simulink model "Mdl_Speed"  (R2024b)
settings: Solver=FixedStepDiscrete  StartTime=0.0  StopTime=10.0  FixedStep=0.1  RelTol=1e-3  EnableMultiTasking=on
values from neighbouring files (symbols this model uses):
  AI_TEMP_ADC_COUNT_1586 = mpt.Parameter    [Mdl_Speed_lookup.m]
  AI_TEMP_ADC_COUNT_1727 = mpt.Parameter    [Mdl_Speed_lookup.m]
  AI_TEMP_ADC_COUNT_1792 = mpt.Parameter    [Mdl_Speed_lookup.m]
  AI_TEMP_ADC_COUNT_1891 = mpt.Parameter    [Mdl_Speed_lookup.m]
  C_ADR = mpt.Parameter    [Mdl_Speed_lookup.m]
  C_CANADA = mpt.Parameter    [Mdl_Speed_lookup.m]
  C_EUROPE = mpt.Parameter    [Mdl_Speed_lookup.m]
  C_KOREA = mpt.Parameter    [Mdl_Speed_lookup.m]
  C_MEXICO = mpt.Parameter    [Mdl_Speed_lookup.m]
  C_UK = mpt.Parameter    [Mdl_Speed_lookup.m]
  C_USA = mpt.Parameter    [Mdl_Speed_lookup.m]
  eSP_ADR = mpt.Parameter    [Speed_Table_Type_param.m]
  eSP_CANADA = mpt.Parameter    [Speed_Table_Type_param.m]
  eSP_ECE = mpt.Parameter    [Speed_Table_Type_param.m]
  eSP_EUROPE = mpt.Parameter    [Speed_Table_Type_param.m]
  eSP_KOREA_FMVSS = mpt.Parameter    [Speed_Table_Type_param.m]
  eSP_KOREA_UN_R = mpt.Parameter    [Speed_Table_Type_param.m]
  eSP_MEXICO_FMVSS = mpt.Parameter    [Speed_Table_Type_param.m]
  eSP_MEXICO_UN_R = mpt.Parameter    [Speed_Table_Type_param.m]
  eSP_UK = mpt.Parameter    [Speed_Table_Type_param.m]
  eSP_USA = mpt.Parameter    [Speed_Table_Type_param.m]
  INDEX_MCUID0262 = mpt.Parameter    [Mdl_Speed_lookup.m]
  INDEX_MCUID0263 = mpt.Parameter    [Mdl_Speed_lookup.m]
  Initial_data = mpt.Parameter    [Mdl_Speed_lookup.m]
  MCUID0809 = mpt.Parameter    [Mdl_Speed_DD.m]
  MCUID0810 = mpt.Parameter    [Mdl_Speed_DD.m]
  MCUID_MAX_VAL = mpt.Parameter    [Mdl_Speed_lookup.m]
  MIN_SPEED_VALUE = mpt.Parameter    [Mdl_Speed_lookup.m]
  RESOLUTION_VAL_100 = mpt.Parameter    [Mdl_Speed_lookup.m]
  RESOLUTION_VAL_103 = mpt.Parameter    [Mdl_Speed_lookup.m]
  RESOLUTION_VAL_50 = mpt.Parameter    [Mdl_Speed_lookup.m]
  RESOLUTION_VAL_64 = mpt.Parameter    [Mdl_Speed_lookup.m]
  RESOLUTION_VAL_MINUS_100 = mpt.Parameter    [Mdl_Speed_lookup.m]
  SPEED_AVG_REF = mpt.Parameter    [Mdl_Speed_lookup.m]
  SPEED_CHECK_VALUE_ONE = mpt.Parameter    [Mdl_Speed_lookup.m]
  SPEED_UPDATE_0_28S = mpt.Parameter    [Mdl_Speed_lookup.m]
  SPEED_UPDATE_0_5S = mpt.Parameter    [Mdl_Speed_lookup.m]
  SPEED_UPDATE_1_5S = mpt.Parameter    [Mdl_Speed_lookup.m]
  SPEED_UPDATE_1S = mpt.Parameter    [Mdl_Speed_lookup.m]
  SPEED_ZERO = mpt.Parameter    [Mdl_Speed_lookup.m]
  VAL_ONE = mpt.Parameter    [Mdl_Speed_lookup.m]
  VAL_ZERO = mpt.Parameter    [Mdl_Speed_lookup.m]
undefined symbols (not defined in the file or in its folder): Arr_u8_100_type_instance, Arr_u8_1024_type_instance, Arr_u8_10_type_instance, Arr_u8_128_type_instance, Arr_u8_16_type_instance, Arr_u8_17_type_instance, Arr_u8_2048_type_instance, Arr_u8_256_type_instance, Arr_u8_32_type_instance, Arr_u8_3_type_instance, Arr_u8_46_type_instance, Arr_u8_48_type_instance, Arr_u8_61_type_instance, Arr_u8_64_type_instance, Arr_u8_8_type_instance, Arr_u8_9_type_instance, CLUSTER_ACTIVE, eIO_ADC_AI_TEMP_RTC, eSIGNAL_MISSING, eSIGNAL_NEVER_RECEIVED, eVehicleSpeedABSIn, IgnOff, IgnOn, IoHwAb_AdcSignalIdType_type_instance, IoHwAb_ErrorType_type_instance, pJustRcvdStatus, RxCan_SignalClearJustRcvdStatus, RxCan_SignalGetJustRcvdStatus, RxCan_SignalInvalidProcessingControl, RxCan_SignalMissingProcessingControl, RxCan_SignalNRProcessingControl, SignalId, SPEED_MAX_RESOLUTION, Status, tRxSignalId_type_instance, tRxSignalJustRcvdStatus_type_instance, tRxSignalStatus_type_instance
libraries: simulink x9
(part 1 of 3)
settings Model: Creator=AELANGO6  LastModifiedBy=AELANGO6
settings DataIOCC: SaveOutput=off
settings OptimizationCC: DefaultParameterBehavior=Inlined  EnhancedBackFolding=on  PassReuseOutputArgsAs=Individual arguments  ZeroExternalMemoryAtStartup=off  ZeroInternalMemoryAtStartup=off  MaxStackSize=750  OptimizeBlockOrder=speed  DifferentSizesBufferReuse=on  OptimizationCustomize=off  EfficientTunableParamExpr=on
settings DebuggingCC: ParameterTunabilityLossMsg=error
settings SFSimCC: MATLABDynamicMemAlloc=off
settings RTWCC: Description=AUTOSAR  SystemTargetFile=autosar.tlc  GenCodeOnly=on  TemplateMakefile=ert_default_tmf  PortableWordSizes=on  DataTypeReplacement=CDataTypesFixedWidth
settings CodeAppCC: ForceParamTrailComments=on  IgnoreCustomStorageClasses=off  OperatorAnnotations=on  SimulinkDataObjDesc=on  SFDataObjDesc=on  InsertBlockDesc=on
settings STFCustomTargetCC: TargetLangStandard=C99 (ISO)  MultiwordLength=256  ParMdlRefBuildCompliant=on  CompOptLevelCompliant=on  IncludeMdlTerminateFcn=off  CombineOutputUpdateFcns=on  SuppressErrorStatus=on  ERTCustomFileBanners=on  SupportNonFinite=off  SupportComplex=off  SupportContinuousTime=off  SupportNonInlinedSFcns=off  RemoveResetFunc=on  ParenthesesLevel=Maximum  CastingMode=Standards  MATLABClassNameForMDSCustomization=Simulink.SoftwareTarget.ERTCustomization  AutosarCompliant=on  UseToolchainInfoCompliant=on  LookupTableObjectStructAxisOrder=2,1,3,4,...  LUTObjectStructOrderEvenSpacing=Size,Table,Breakpoints  SystemTargetFile=autosar.tlc
settings ERTTargetCC: TargetLangStandard=C99 (ISO)  ConcurrentExecutionCompliant=off  IncludeMdlTerminateFcn=off  SuppressErrorStatus=on  SupportNonFinite=off  SupportComplex=off  ParenthesesLevel=Maximum  CastingMode=Standards  ModelStepFunctionPrototypeControlCompliant=off  CPPClassGenCompliant=off  AutosarCompliant=on  LookupTableObjectStructAxisOrder=2,1,3,4,...  LUTObjectStructOrderEvenSpacing=Size,Table,Breakpoints  ERTCustomFileTemplate=example_file_process.tlc  ERTFilePackagingFormat=CompactWithDataFile  BooleanTrueId=TRUE  BooleanFalseId=FALSE

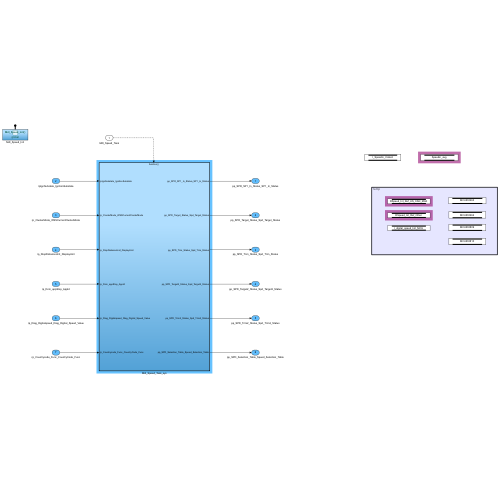
[thumbnail: Simulink's stored preview of the top-level diagram]
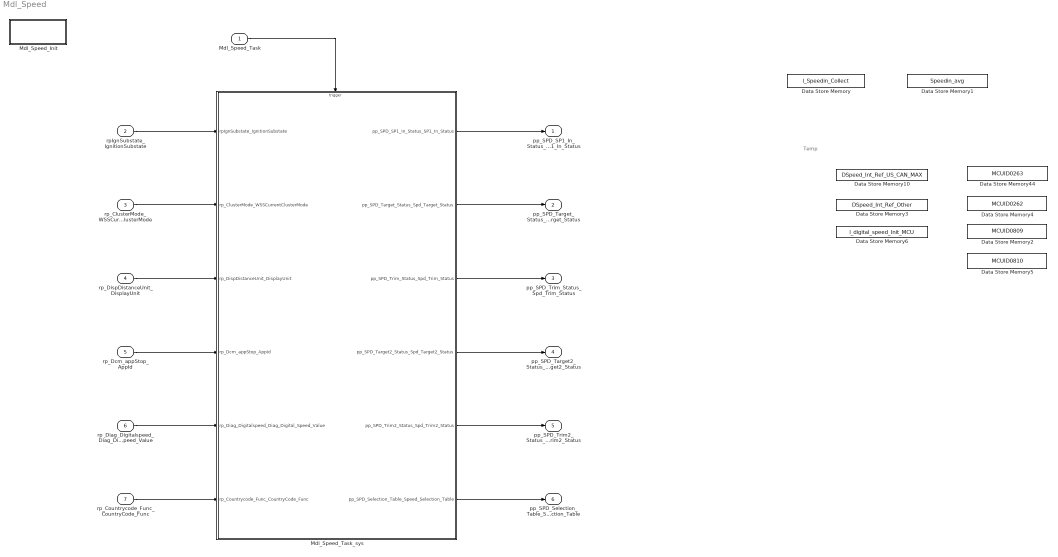
== system Mdl_Speed ==
  note: Temp
  Mdl_Speed_Task : Inport  SampleTime=0.1  OutputFunctionCall=on
  rpIgnSubstate_IgnitionSubstate : Inport  Port=2  OutDataTypeStr=IgntionSubstateType  PortDimensions=1
  rp_ClusterMode_WSSCurrentClusterMode : Inport  Port=3  OutDataTypeStr=ClusterModes  PortDimensions=1
  rp_DispDistanceUnit_DisplayUnit : Inport  Port=4  OutDataTypeStr=uint8  PortDimensions=1
  rp_Dcm_appStop_AppId : Inport  Port=5  OutDataTypeStr=IOCtrl_Type  PortDimensions=1
  rp_Diag_Digitalspeed_Diag_Digital_Speed_Value : Inport  Port=6  OutDataTypeStr=uint16  PortDimensions=1
  rp_Countrycode_Func_CountryCode_Func : Inport  Port=7  OutDataTypeStr=CountryCode_FuncType  PortDimensions=1
  Data Store Memory : DataStoreMemory  DataStoreName=l_Speedin_Collect  ReadBeforeWriteMsg=warning  WriteAfterWriteMsg=warning  WriteAfterReadMsg=warning  ShowAdditionalParam=off  OutDataTypeStr=uint32
  Data Store Memory1 : DataStoreMemory  DataStoreName=Speedin_avg  ReadBeforeWriteMsg=warning  WriteAfterWriteMsg=warning  WriteAfterReadMsg=warning  ShowAdditionalParam=off  OutDataTypeStr=uint16
  Data Store Memory10 : DataStoreMemory  DataStoreName=DSpeed_Int_Ref_US_CAN_MAX  ReadBeforeWriteMsg=warning  WriteAfterWriteMsg=warning  WriteAfterReadMsg=warning  InitialValue=Initial_data  ShowAdditionalParam=off  OutDataTypeStr=uint16  Dimensions=21
  Data Store Memory2 : DataStoreMemory  DataStoreName=MCUID0809  ReadBeforeWriteMsg=warning  WriteAfterWriteMsg=warning  WriteAfterReadMsg=warning  InitialValue=VAL_ZERO  ShowAdditionalParam=off  OutDataTypeStr=uint8
  Data Store Memory3 : DataStoreMemory  DataStoreName=DSpeed_Int_Ref_Other  ReadBeforeWriteMsg=warning  WriteAfterWriteMsg=warning  WriteAfterReadMsg=warning  InitialValue=Initial_data  ShowAdditionalParam=off  OutDataTypeStr=uint16  Dimensions=21
  Data Store Memory4 : DataStoreMemory  DataStoreName=MCUID0262  ReadBeforeWriteMsg=warning  WriteAfterWriteMsg=warning  WriteAfterReadMsg=warning  InitialValue=CNVM_MCUID0262_DEFAULT_VAL  ShowAdditionalParam=off  OutDataTypeStr=uint16
  Data Store Memory44 : DataStoreMemory  DataStoreName=MCUID0263  ReadBeforeWriteMsg=warning  WriteAfterWriteMsg=warning  WriteAfterReadMsg=warning  InitialValue=CNVM_MCUID0263_DEFAULT_VAL  ShowAdditionalParam=off  OutDataTypeStr=uint16
  Data Store Memory5 : DataStoreMemory  DataStoreName=MCUID0810  ReadBeforeWriteMsg=warning  WriteAfterWriteMsg=warning  WriteAfterReadMsg=warning  InitialValue=VAL_ONE  ShowAdditionalParam=off  OutDataTypeStr=uint8
  Data Store Memory6 : DataStoreMemory  DataStoreName=l_digital_speed_Init_MCU  ReadBeforeWriteMsg=warning  WriteAfterWriteMsg=warning  WriteAfterReadMsg=warning  InitialValue=VAL_ZERO  ShowAdditionalParam=off  OutDataTypeStr=uint8
  Mdl_Speed_Init : Subsystem  TreatAsAtomicUnit=on
  Mdl_Speed_Task_sys : Subsystem  TreatAsAtomicUnit=on
  pp_SPD_SP1_In_Status_SP1_In_Status : Outport  OutDataTypeStr=uint16
  pp_SPD_Target_Status_Spd_Target_Status : Outport  Port=2  OutDataTypeStr=uint16
  pp_SPD_Trim_Status_Spd_Trim_Status : Outport  Port=3  OutDataTypeStr=uint16
  pp_SPD_Target2_Status_Spd_Target2_Status : Outport  Port=4  OutDataTypeStr=uint16
  pp_SPD_Trim2_Status_Spd_Trim2_Status : Outport  Port=5  OutDataTypeStr=uint16
  pp_SPD_Selection_Table_Speed_Selection_Table : Outport  Port=6  OutDataTypeStr=uint8
  wires:
  rp_Countrycode_Func_CountryCode_Func/1 -> Mdl_Speed_Task_sys/6(rp_Countrycode_Func_CountryCode_Func)
  rpIgnSubstate_IgnitionSubstate/1 -> Mdl_Speed_Task_sys/1(rpIgnSubstate_IgnitionSubstate)
  Mdl_Speed_Task/1 -> Mdl_Speed_Task_sys/Trigger
  rp_ClusterMode_WSSCurrentClusterMode/1 -> Mdl_Speed_Task_sys/2(rp_ClusterMode_WSSCurrentClusterMode)
  rp_DispDistanceUnit_DisplayUnit/1 -> Mdl_Speed_Task_sys/3(rp_DispDistanceUnit_DisplayUnit)
  rp_Dcm_appStop_AppId/1 -> Mdl_Speed_Task_sys/4(rp_Dcm_appStop_AppId)
  rp_Diag_Digitalspeed_Diag_Digital_Speed_Value/1 -> Mdl_Speed_Task_sys/5(rp_Diag_Digitalspeed_Diag_Digital_Speed_Value)
  Mdl_Speed_Task_sys/1(pp_SPD_SP1_In_Status_SP1_In_Status) -> pp_SPD_SP1_In_Status_SP1_In_Status/1
  Mdl_Speed_Task_sys/2(pp_SPD_Target_Status_Spd_Target_Status) -> pp_SPD_Target_Status_Spd_Target_Status/1
  Mdl_Speed_Task_sys/3(pp_SPD_Trim_Status_Spd_Trim_Status) -> pp_SPD_Trim_Status_Spd_Trim_Status/1
  Mdl_Speed_Task_sys/4(pp_SPD_Target2_Status_Spd_Target2_Status) -> pp_SPD_Target2_Status_Spd_Target2_Status/1
  Mdl_Speed_Task_sys/5(pp_SPD_Trim2_Status_Spd_Trim2_Status) -> pp_SPD_Trim2_Status_Spd_Trim2_Status/1
  Mdl_Speed_Task_sys/6(pp_SPD_Selection_Table_Speed_Selection_Table) -> pp_SPD_Selection_Table_Speed_Selection_Table/1

== system Mdl_Speed/Mdl_Speed_Init ==
  Mdl_Speed_Init : TriggerPort  TriggerType=function-call  IsSimulinkFunction=on  FunctionName=Mdl_Speed_Init  VariantControl=(inherit)

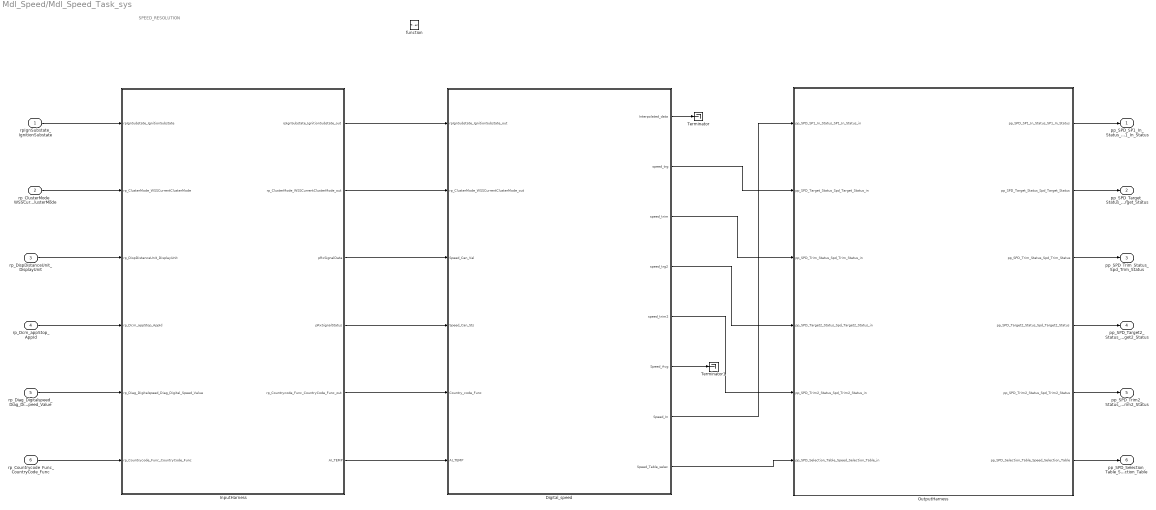
== system Mdl_Speed/Mdl_Speed_Task_sys ==
  note: SPEED_RESOLUTION
  rpIgnSubstate_IgnitionSubstate : Inport  OutDataTypeStr=IgntionSubstateType  PortDimensions=1
  rp_ClusterMode_WSSCurrentClusterMode : Inport  Port=2  OutDataTypeStr=ClusterModes  PortDimensions=1
  rp_DispDistanceUnit_DisplayUnit : Inport  Port=3  OutDataTypeStr=uint8  PortDimensions=1
  rp_Dcm_appStop_AppId : Inport  Port=4  OutDataTypeStr=IOCtrl_Type  PortDimensions=1
  rp_Diag_Digitalspeed_Diag_Digital_Speed_Value : Inport  Port=5  OutDataTypeStr=uint16  PortDimensions=1
  rp_Countrycode_Func_CountryCode_Func : Inport  Port=6  OutDataTypeStr=CountryCode_FuncType  PortDimensions=1
  function : TriggerPort  TriggerType=function-call  VariantControl=(inherit)  SampleTimeType=periodic  SampleTime=-1
  Digital_speed : Subsystem
  InputHarness : Subsystem  Variant=on
  OutputHarness : Subsystem  Variant=on
  Terminator : Terminator
  Terminator1 : Terminator
  pp_SPD_SP1_In_Status_SP1_In_Status : Outport  OutDataTypeStr=uint16  PortDimensions=1
  pp_SPD_Target_Status_Spd_Target_Status : Outport  Port=2  OutDataTypeStr=uint16  PortDimensions=1
  pp_SPD_Trim_Status_Spd_Trim_Status : Outport  Port=3  OutDataTypeStr=uint16  PortDimensions=1
  pp_SPD_Target2_Status_Spd_Target2_Status : Outport  Port=4  OutDataTypeStr=uint16  PortDimensions=1
  pp_SPD_Trim2_Status_Spd_Trim2_Status : Outport  Port=5  OutDataTypeStr=uint16  PortDimensions=1
  pp_SPD_Selection_Table_Speed_Selection_Table : Outport  Port=6  OutDataTypeStr=uint8  PortDimensions=1
  wires:
  rp_Countrycode_Func_CountryCode_Func/1 -> InputHarness/6(rp_Countrycode_Func_CountryCode_Func)
  rpIgnSubstate_IgnitionSubstate/1 -> InputHarness/1(rpIgnSubstate_IgnitionSubstate)
  rp_ClusterMode_WSSCurrentClusterMode/1 -> InputHarness/2(rp_ClusterMode_WSSCurrentClusterMode)
  rp_DispDistanceUnit_DisplayUnit/1 -> InputHarness/3(rp_DispDistanceUnit_DisplayUnit)
  rp_Dcm_appStop_AppId/1 -> InputHarness/4(rp_Dcm_appStop_AppId)
  rp_Diag_Digitalspeed_Diag_Digital_Speed_Value/1 -> InputHarness/5(rp_Diag_Digitalspeed_Diag_Digital_Speed_Value)
  OutputHarness/1(pp_SPD_SP1_In_Status_SP1_In_Status) -> pp_SPD_SP1_In_Status_SP1_In_Status/1
  OutputHarness/2(pp_SPD_Target_Status_Spd_Target_Status) -> pp_SPD_Target_Status_Spd_Target_Status/1
  OutputHarness/3(pp_SPD_Trim_Status_Spd_Trim_Status) -> pp_SPD_Trim_Status_Spd_Trim_Status/1
  OutputHarness/4(pp_SPD_Target2_Status_Spd_Target2_Status) -> pp_SPD_Target2_Status_Spd_Target2_Status/1
  OutputHarness/5(pp_SPD_Trim2_Status_Spd_Trim2_Status) -> pp_SPD_Trim2_Status_Spd_Trim2_Status/1
  OutputHarness/6(pp_SPD_Selection_Table_Speed_Selection_Table) -> pp_SPD_Selection_Table_Speed_Selection_Table/1
  InputHarness/1(rpIgnSubstate_IgnitionSubstate_out) -> Digital_speed/1(rpIgnSubstate_IgnitionSubstate_out)
  InputHarness/2(rp_ClusterMode_WSSCurrentClusterMode_out) -> Digital_speed/2(rp_ClusterMode_WSSCurrentClusterMode_out)
  InputHarness/3(pRxSignalData) -> Digital_speed/3(Speed_Can_Val)
  InputHarness/4(pRxSignalStatus) -> Digital_speed/4(Speed_Can_Sts)
  InputHarness/6(AI_TEMP) -> Digital_speed/6(AI_TEMP)
  InputHarness/5(rp_Countrycode_Func_CountryCode_Func_out) -> Digital_speed/5(Country_code_Func)
  Digital_speed/2(speed_trg) -> OutputHarness/2(pp_SPD_Target_Status_Spd_Target_Status_in)
  Digital_speed/1(Interpolated_data) -> Terminator/1
  Digital_speed/6(Speed_Avg) -> Terminator1/1
  Digital_speed/3(speed_trim) -> OutputHarness/3(pp_SPD_Trim_Status_Spd_Trim_Status_in)
  Digital_speed/4(speed_trg2) -> OutputHarness/4(pp_SPD_Target2_Status_Spd_Target2_Status_in)
  Digital_speed/5(speed_trim2) -> OutputHarness/5(pp_SPD_Trim2_Status_Spd_Trim2_Status_in)
  Digital_speed/7(Speed_In) -> OutputHarness/1(pp_SPD_SP1_In_Status_SP1_In_Status_in)
  Digital_speed/8(Speed_Table_selec) -> OutputHarness/6(pp_SPD_Selection_Table_Speed_Selection_Table_in)

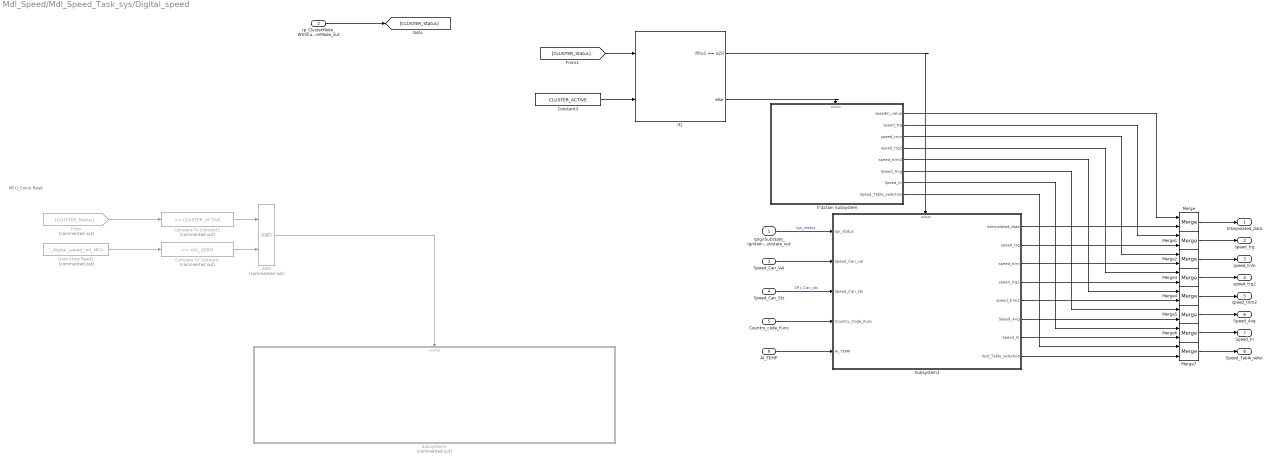
== system Mdl_Speed/Mdl_Speed_Task_sys/Digital_speed ==
  note: MCU_Const Read
  rpIgnSubstate_IgnitionSubstate_out : Inport  OutDataTypeStr=IgntionSubstateType  PortDimensions=1
  rp_ClusterMode_WSSCurrentClusterMode_out : Inport  Port=2
  Speed_Can_Val : Inport  Port=3  OutDataTypeStr=uint8
  Speed_Can_Sts : Inport  Port=4  OutDataTypeStr=uint8
  Country_code_Func : Inport  Port=5  OutDataTypeStr=uint8
  AI_TEMP : Inport  Port=6
  AND : Logic  Commented=on  AllPortsSameDT=off  OutDataTypeStr=boolean
  Compare To Constant : simulink/Logic and Bit Operations/Compare To Constant  Commented=on  relop===  const=VAL_ZERO  OutDataTypeStr=boolean
  Compare To Constant1 : simulink/Logic and Bit Operations/Compare To Constant  Commented=on  relop===  const=CLUSTER_ACTIVE  OutDataTypeStr=boolean
  Constant3 : Constant  Value=CLUSTER_ACTIVE
  Data Store Read2 : DataStoreRead  Commented=on  DataStoreName=l_digital_speed_Init_MCU  IndexOptions=Index vector (dialog)  Indices=1  OutputSizes=1
  From : From  Commented=on  GotoTag=CLUSTER_Status
  If Action Subsystem : Subsystem  TreatAsAtomicUnit=on
  If1 : If  NumInputs=2  IfExpression=(u1 == u2)
  Merge{,1..7} (8 alike) : Merge
  Subsystem1 : Subsystem
  Subsystem2 : Subsystem  Commented=on  RTWFcnName=MCUConst_Read
      settings: RTWSystemCode=Nonreusable function  RTWFcnNameOpts=User specified  FunctionInterfaceSpec=Allow arguments (Optimized)
  Interpolated_data : Outport  OutDataTypeStr=uint16  VectorParamsAs1DForOutWhenUnconnected=off
  speed_trg : Outport  Port=2  OutDataTypeStr=uint16  VectorParamsAs1DForOutWhenUnconnected=off
  speed_trim : Outport  Port=3  OutDataTypeStr=uint16  VectorParamsAs1DForOutWhenUnconnected=off
  speed_trg2 : Outport  Port=4  OutDataTypeStr=uint16  VectorParamsAs1DForOutWhenUnconnected=off
  speed_trim2 : Outport  Port=5  OutDataTypeStr=uint16  VectorParamsAs1DForOutWhenUnconnected=off
  Speed_Avg : Outport  Port=6  OutDataTypeStr=uint16  VectorParamsAs1DForOutWhenUnconnected=off
  Speed_In : Outport  Port=7  VectorParamsAs1DForOutWhenUnconnected=off
  Speed_Table_selec : Outport  Port=8  VectorParamsAs1DForOutWhenUnconnected=off
  wires:
  Speed_Can_Sts/1 -> Subsystem1/3(Speed_Can_sts)  "SP1_Can_sts"
  rpIgnSubstate_IgnitionSubstate_out/1 -> Subsystem1/1(Ign_status)  "Ign_status"
  Speed_Can_Val/1 -> Subsystem1/2(Speed_Can_val)
  If1/1 -> Subsystem1/Action
  If1/2 -> If Action Subsystem/Action
  If Action Subsystem/1(speedIn_value) -> Merge/1
  Subsystem1/1(Interpolated_data) -> Merge/2
  Merge/1 -> Interpolated_data/1
  Subsystem1/2(speed_trg) -> Merge1/2
  Merge1/1 -> speed_trg/1
  If Action Subsystem/2(speed_trg) -> Merge1/1
  Merge2/1 -> speed_trim/1
  Subsystem1/3(speed_trim) -> Merge2/2
  If Action Subsystem/3(speed_trim) -> Merge2/1
  Merge4/1 -> speed_trim2/1
  Merge3/1 -> speed_trg2/1
  Subsystem1/4(speed_trg2) -> Merge3/2
  Subsystem1/5(speed_trim2) -> Merge4/2
  If Action Subsystem/4(speed_trg2) -> Merge3/1
  If Action Subsystem/5(speed_trim2) -> Merge4/1
  Country_code_Func/1 -> Subsystem1/4(Country_Code_Func)
  AI_TEMP/1 -> Subsystem1/5(AI_TEMP)
  Merge5/1 -> Speed_Avg/1
  Subsystem1/6(Speed_Avg) -> Merge5/2
  If Action Subsystem/6(Speed_Avg) -> Merge5/1
  Subsystem1/7(Speed_In) -> Merge6/2
  If Action Subsystem/7(Speed_In) -> Merge6/1
  Merge6/1 -> Speed_In/1
  If Action Subsystem/8(Speed_Table_selection) -> Merge7/1
  Subsystem1/8(Spd_Table_selection) -> Merge7/2
  Merge7/1 -> Speed_Table_selec/1
  Data Store Read2/1 -> Compare To Constant/1
  Compare To Constant1/1 -> AND/1
  AND/1 -> Subsystem2/Enable
  Compare To Constant/1 -> AND/2
  From/1 -> Compare To Constant1/1
  Constant3/1 -> If1/2
  [CLUSTER_Status] -> If1/1
  rp_ClusterMode_WSSCurrentClusterMode_out/1 -> [CLUSTER_Status]

== system Mdl_Speed/Mdl_Speed_Task_sys/InputHarness ==
  rpIgnSubstate_IgnitionSubstate : Inport  OutDataTypeStr=IgntionSubstateType  PortDimensions=1
  rp_ClusterMode_WSSCurrentClusterMode : Inport  Port=2  OutDataTypeStr=ClusterModes  PortDimensions=1
  rp_DispDistanceUnit_DisplayUnit : Inport  Port=3  OutDataTypeStr=uint8  PortDimensions=1
  rp_Dcm_appStop_AppId : Inport  Port=4  OutDataTypeStr=IOCtrl_Type  PortDimensions=1
  rp_Diag_Digitalspeed_Diag_Digital_Speed_Value : Inport  Port=5  OutDataTypeStr=uint16  PortDimensions=1
  rp_Countrycode_Func_CountryCode_Func : Inport  Port=6  OutDataTypeStr=CountryCode_FuncType  PortDimensions=1
  CodeGeneration : Subsystem  VariantControl=CODEGENERATION
  Simulation : Subsystem  VariantControl=SIMULATION
  rpIgnSubstate_IgnitionSubstate_out : Outport  OutDataTypeStr=IgntionSubstateType  PortDimensions=1
  rp_ClusterMode_WSSCurrentClusterMode_out : Outport  Port=2  OutDataTypeStr=ClusterModes  PortDimensions=1
  pRxSignalData : Outport  Port=3  OutDataTypeStr=uint8  VectorParamsAs1DForOutWhenUnconnected=off
  pRxSignalStatus : Outport  Port=4  OutDataTypeStr=uint8  VectorParamsAs1DForOutWhenUnconnected=off
  rp_Countrycode_Func_CountryCode_Func_out : Outport  Port=5  OutDataTypeStr=CountryCode_FuncType  PortDimensions=1
  AI_TEMP : Outport  Port=6  VectorParamsAs1DForOutWhenUnconnected=off

== system Mdl_Speed/Mdl_Speed_Task_sys/OutputHarness ==
  pp_SPD_SP1_In_Status_SP1_In_Status_in : Inport  OutDataTypeStr=uint16  PortDimensions=1
  pp_SPD_Target_Status_Spd_Target_Status_in : Inport  Port=2  OutDataTypeStr=uint16  PortDimensions=1
  pp_SPD_Trim_Status_Spd_Trim_Status_in : Inport  Port=3  OutDataTypeStr=uint16  PortDimensions=1
  pp_SPD_Target2_Status_Spd_Target2_Status_in : Inport  Port=4  OutDataTypeStr=uint16  PortDimensions=1
  pp_SPD_Trim2_Status_Spd_Trim2_Status_in : Inport  Port=5  OutDataTypeStr=uint16  PortDimensions=1
  pp_SPD_Selection_Table_Speed_Selection_Table_in : Inport  Port=6  OutDataTypeStr=uint8  PortDimensions=1
  CodeGeneration : Subsystem  VariantControl=CODEGENERATION
  Simulation : Subsystem  VariantControl=SIMULATION
  pp_SPD_SP1_In_Status_SP1_In_Status : Outport  OutDataTypeStr=uint16  PortDimensions=1
  pp_SPD_Target_Status_Spd_Target_Status : Outport  Port=2  OutDataTypeStr=uint16  PortDimensions=1
  pp_SPD_Trim_Status_Spd_Trim_Status : Outport  Port=3  OutDataTypeStr=uint16  PortDimensions=1
  pp_SPD_Target2_Status_Spd_Target2_Status : Outport  Port=4  OutDataTypeStr=uint16  PortDimensions=1
  pp_SPD_Trim2_Status_Spd_Trim2_Status : Outport  Port=5  OutDataTypeStr=uint16  PortDimensions=1
  pp_SPD_Selection_Table_Speed_Selection_Table : Outport  Port=6  OutDataTypeStr=uint8  PortDimensions=1

== system Mdl_Speed/Mdl_Speed_Task_sys/Digital_speed/If Action Subsystem ==
  Action Port : ActionPort  ActionPortLabel=else
  Constant : Constant  Value=SPEED_ZERO  SampleTime=-1
  Constant1 : Constant  Value=VAL_ZERO  OutDataTypeStr=uint8  SampleTime=-1
  speedIn_value : Outport  OutDataTypeStr=uint16  VectorParamsAs1DForOutWhenUnconnected=off
  speed_trg : Outport  Port=2  OutDataTypeStr=uint16  VectorParamsAs1DForOutWhenUnconnected=off
  speed_trim : Outport  Port=3  OutDataTypeStr=uint16  VectorParamsAs1DForOutWhenUnconnected=off
  speed_trg2 : Outport  Port=4  OutDataTypeStr=uint16  VectorParamsAs1DForOutWhenUnconnected=off
  speed_trim2 : Outport  Port=5  OutDataTypeStr=uint16  VectorParamsAs1DForOutWhenUnconnected=off
  Speed_Avg : Outport  Port=6  VectorParamsAs1DForOutWhenUnconnected=off
  Speed_In : Outport  Port=7  VectorParamsAs1DForOutWhenUnconnected=off
  Speed_Table_selection : Outport  Port=8  OutDataTypeStr=uint8  VectorParamsAs1DForOutWhenUnconnected=off
  wires:
  Constant/1 -> speed_trg2/1, Speed_In/1, Speed_Avg/1, speed_trim2/1, speed_trim/1, speed_trg/1, speedIn_value/1
  Constant1/1 -> Speed_Table_selection/1

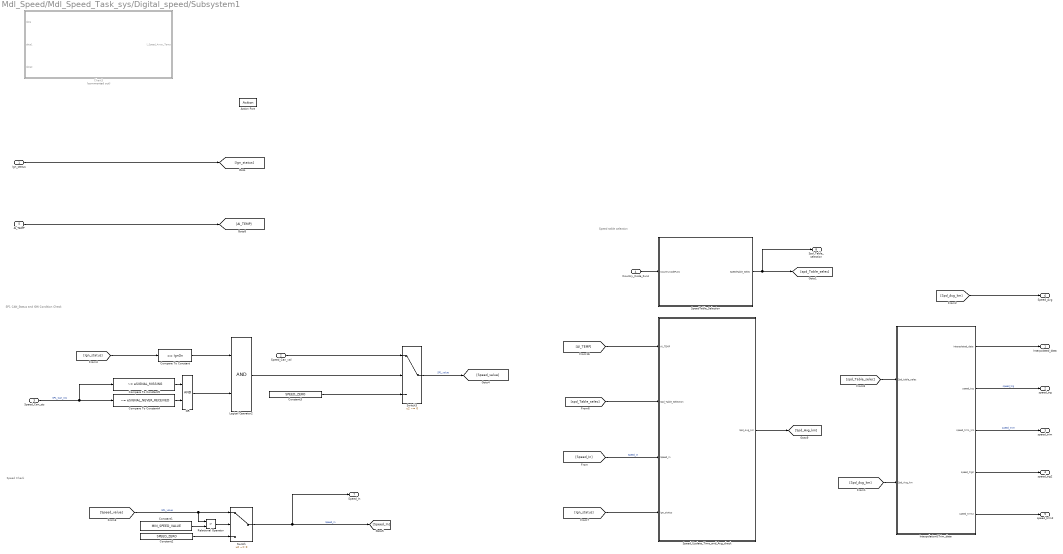
== system Mdl_Speed/Mdl_Speed_Task_sys/Digital_speed/Subsystem1 ==
  note: Speed table selection
  note: SP1 CAN_Status and IGN Condition Check
  note: Speed Check
  Ign_status : Inport
  Speed_Can_val : Inport  Port=2  OutDataTypeStr=uint8
  Speed_Can_sts : Inport  Port=3
  Country_Code_Func : Inport  Port=4  OutDataTypeStr=uint8
  AI_TEMP : Inport  Port=5
  Action Port : ActionPort  ActionPortLabel=if((u1 == u2))
  Chart3 : Stateflow chart  Commented=on  TreatAsAtomicUnit=on  RTWFcnName=Split_NVM_Speed_Ref
      settings: RTWSystemCode=Reusable function  RTWFcnNameOpts=User specified
  Compare To Constant : simulink/Logic and Bit Operations/Compare To Constant  relop===  const=IgnOn  OutDataTypeStr=boolean
  Compare To Constant4 : simulink/Logic and Bit Operations/Compare To Constant  relop=~=  const=eSIGNAL_NEVER_RECEIVED  OutDataTypeStr=boolean
  Compare To Constant5 : simulink/Logic and Bit Operations/Compare To Constant  relop=~=  const=eSIGNAL_MISSING  OutDataTypeStr=boolean
  Constant1 : Constant  Value=MIN_SPEED_VALUE  OutDataTypeStr=uint16
  Constant2 : Constant  Value=SPEED_ZERO  OutDataTypeStr=uint16
  Constant3 : Constant  Value=SPEED_ZERO  OutDataTypeStr=uint16
  Interpolation&Trim_data : Subsystem
  Logical Operator2 : Logic  AllPortsSameDT=off  OutDataTypeStr=boolean
  OR : Logic  AllPortsSameDT=off  OutDataTypeStr=boolean
  Relational Operator : RelationalOperator  Operator=>  OutDataTypeStr=boolean  RndMeth=Simplest  InputSameDT=off
  SpeedTable_Selection : Subsystem
  Speed_Update_Time_and_Avg_check : Subsystem
  Switch : Switch  Criteria=u2 ~= 0  RndMeth=Simplest  SaturateOnIntegerOverflow=off  InputSameDT=off
  Switch3 : Switch  Criteria=u2 ~= 0  RndMeth=Simplest  SaturateOnIntegerOverflow=off  InputSameDT=off
  Interpolated_data : Outport  OutDataTypeStr=uint16  VectorParamsAs1DForOutWhenUnconnected=off
  speed_trg : Outport  Port=2  OutDataTypeStr=uint16  VectorParamsAs1DForOutWhenUnconnected=off
  speed_trim : Outport  Port=3  OutDataTypeStr=uint16  VectorParamsAs1DForOutWhenUnconnected=off
  speed_trg2 : Outport  Port=4  OutDataTypeStr=uint16  VectorParamsAs1DForOutWhenUnconnected=off
  speed_trim2 : Outport  Port=5  OutDataTypeStr=uint16  VectorParamsAs1DForOutWhenUnconnected=off
  Speed_Avg : Outport  Port=6  OutDataTypeStr=uint16  VectorParamsAs1DForOutWhenUnconnected=off
  Speed_In : Outport  Port=7  VectorParamsAs1DForOutWhenUnconnected=off
  Spd_Table_selection : Outport  Port=8  OutDataTypeStr=uint8  VectorParamsAs1DForOutWhenUnconnected=off
  wires:
  Speed_Can_sts/1 -> Compare To Constant5/1, Compare To Constant4/1  "SP1_Can_sts"
  Switch3/1 -> [Speed_value]  "SP1_value"
  [Speed_value] -> Relational Operator/1, Switch/1  "SP1_value"
  Interpolation&Trim_data/2(speed_trg) -> speed_trg/1  "speed_trg"
  Constant3/1 -> Switch3/3
  Interpolation&Trim_data/3(speed_trim_km) -> speed_trim/1  "speed_trim"
  Relational Operator/1 -> Switch/2
  Switch/1 -> Speed_In/1, [Speed_In]  "Speed_In"
  Logical Operator2/1 -> Switch3/2
  Compare To Constant/1 -> Logical Operator2/1
  Constant2/1 -> Switch/3
  Constant1/1 -> Relational Operator/2
  [Ign_status] -> Compare To Constant/1
  Speed_Can_val/1 -> Switch3/1
  Ign_status/1 -> [Ign_status]
  AI_TEMP/1 -> [AI_TEMP]
  [AI_TEMP] -> Speed_Update_Time_and_Avg_check/1(AI_TEMP)
  [Speed_In] -> Speed_Update_Time_and_Avg_check/3(Speed_In)  "Speed_In"
  [Ign_status] -> Speed_Update_Time_and_Avg_check/4(Ign_status)
  Speed_Update_Time_and_Avg_check/1(Spd_Avg_km) -> [Spd_Avg_km]
  [Spd_Avg_km] -> Interpolation&Trim_data/2(Spd_Avg_km)
  Compare To Constant5/1 -> OR/1
  Compare To Constant4/1 -> OR/2
  OR/1 -> Logical Operator2/2
  [spd_Table_selec] -> Speed_Update_Time_and_Avg_check/2(Spd_Table_Selection)
  [spd_Table_selec] -> Interpolation&Trim_data/1(Spd_table_selec)
  Interpolation&Trim_data/4(speed_trg2) -> speed_trg2/1
  Interpolation&Trim_data/5(speed_trim2) -> speed_trim2/1
  Interpolation&Trim_data/1(Interpolated_data) -> Interpolated_data/1
  [Spd_Avg_km] -> Speed_Avg/1
  SpeedTable_Selection/1(SpeedTable_Selec) -> Spd_Table_selection/1, [spd_Table_selec]
  Country_Code_Func/1 -> SpeedTable_Selection/1(CountrycodeFunc)

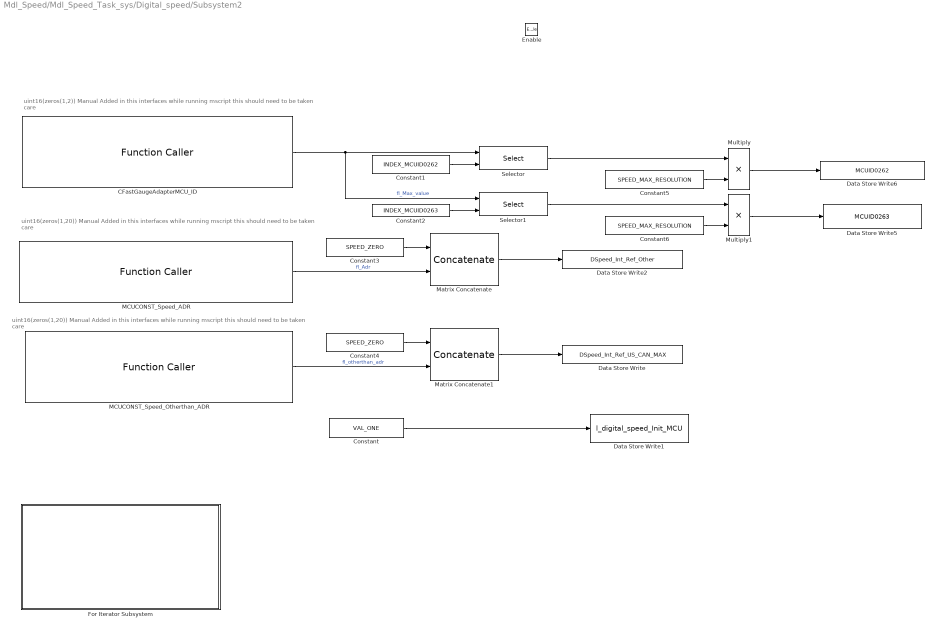
== system Mdl_Speed/Mdl_Speed_Task_sys/Digital_speed/Subsystem2 ==
  note: uint16(zeros(1,20)) Manual Added in this interfaces while running mscript this should need to be taken care
  note: uint16(zeros(1,20)) Manual Added in this interfaces while running mscript this should need to be taken care
  note: uint16(zeros(1,2)) Manual Added in this interfaces while running mscript this should need to be taken care
  Enable : EnablePort
  CFastGaugeAdapterMCU_ID : FunctionCaller  FunctionPrototype=pMCUCONST_Data_FastGauge = CFastGaugeAdapterMCU_ID()  InputArgumentSpecifications=<Enter example>  OutputArgumentSpecifications=uint16(zeros(1,2))
  Constant : Constant  Value=VAL_ONE
  Constant1 : Constant  Value=INDEX_MCUID0262
  Constant2 : Constant  Value=INDEX_MCUID0263
  Constant3 : Constant  Value=SPEED_ZERO  OutDataTypeStr=uint16
  Constant4 : Constant  Value=SPEED_ZERO  OutDataTypeStr=uint16
  Constant5 : Constant  Value=SPEED_MAX_RESOLUTION
  Constant6 : Constant  Value=SPEED_MAX_RESOLUTION
  Data Store Write : DataStoreWrite  DataStoreName=DSpeed_Int_Ref_US_CAN_MAX  IndexOptions=Index vector (dialog)  Indices=1  OutputSizes=1
  Data Store Write1 : DataStoreWrite  DataStoreName=l_digital_speed_Init_MCU  IndexOptions=Index vector (dialog)  Indices=1  OutputSizes=1
  Data Store Write2 : DataStoreWrite  DataStoreName=DSpeed_Int_Ref_Other  IndexOptions=Index vector (dialog)  Indices=1  OutputSizes=1
  Data Store Write5 : DataStoreWrite  DataStoreName=MCUID0263  IndexOptions=Index vector (dialog)  Indices=1  OutputSizes=1
  Data Store Write6 : DataStoreWrite  DataStoreName=MCUID0262  IndexOptions=Index vector (dialog)  Indices=1  OutputSizes=1
  For Iterator Subsystem : Subsystem  TreatAsAtomicUnit=on
  MCUCONST_Speed_ADR : FunctionCaller  FunctionPrototype=pMCUCONST_Speed_Data = MCUCONST_Speed_ADR()  InputArgumentSpecifications=<Enter example>  OutputArgumentSpecifications=uint16(zeros(1,20))
  MCUCONST_Speed_Otherthan_ADR : FunctionCaller  FunctionPrototype=pMCUCONST_Speed_Data = MCUCONST_Speed_Otherthan_ADR()  InputArgumentSpecifications=<Enter example>  OutputArgumentSpecifications=uint16(zeros(1,20))
  Matrix Concatenate : Concatenate
  Matrix Concatenate1 : Concatenate
  Multiply : Product  OutDataTypeStr=uint16
  Multiply1 : Product  OutDataTypeStr=uint16
  Selector : Selector  InputPortWidth=2  IndexOptions=Index vector (port)  Indices=[1 3]  OutputSizes=1
  Selector1 : Selector  InputPortWidth=2  IndexOptions=Index vector (port)  Indices=[1 3]  OutputSizes=1
  wires:
  Constant/1 -> Data Store Write1/1
  CFastGaugeAdapterMCU_ID/1 -> Selector/1, Selector1/1  "fl_Max_value"
  Constant1/1 -> Selector/2
  Constant2/1 -> Selector1/2
  MCUCONST_Speed_ADR/1 -> Matrix Concatenate/2  "fl_Adr"
  Matrix Concatenate/1 -> Data Store Write2/1
  Constant3/1 -> Matrix Concatenate/1
  MCUCONST_Speed_Otherthan_ADR/1 -> Matrix Concatenate1/2  "fl_otherthan_adr"
  Constant4/1 -> Matrix Concatenate1/1
  Matrix Concatenate1/1 -> Data Store Write/1
  Selector1/1 -> Multiply1/1
  Selector/1 -> Multiply/1
  Constant6/1 -> Multiply1/2
  Constant5/1 -> Multiply/2
  Multiply/1 -> Data Store Write6/1
  Multiply1/1 -> Data Store Write5/1
